simulink model "ctc_sim"  (R2019b)
settings: Solver=VariableStepAuto  StartTime=0.0  StopTime=T  FixedStep=0.001  MaxStep=0.01  RelTol=1e-3
values from neighbouring files (symbols this model uses):
  bsc = 17    [model.mat]    (also in model_data.m)
  d_r = [0.01 0.01 0.01 0.01 0.01 0.01]    [model.mat]    (also in model_data.m = 0.01*ones(6,1))
  Fi_b_z = [0 2.09439510239 4.18879020479 1.0471975512 3.14159265359 5.23598775598]    [model.mat]    (also in model_data.m = [0;2/3;4/3;1/3;3/3;5/3]*pi)
  Kd = 0    [ctc_data.m]
  Ki = 0    [ctc_data.m]
  Kp = 300    [ctc_data.m]
  ksc = 179000    [model.mat]    (also in model_data.m)
  l_r = [0.36 0.36 0.36 0.36 0.36 0.36]    [model.mat]    (also in model_data.m = 0.36*ones(6,1))
  linderiv = 0    [model.mat]    (also in model_data.m)
  O_lb = [0 0 0 0 0 0]    [model.mat]    (also in model_data.m = [0;0;0;0;0;0])
  q_d = out_ik.q'    [ik_run.m]
  qt_d = out_ik.qt'    [ik_run.m]
  qtt_d = out_ik.qtt'    [ik_run.m]
  s = out_ctc.s    [ctc_run.m]
  s_0 = s_d(:,:,1)    [ctc_run.m]    (also in iff_run.m)
  t_d = out_ik.t'    [ik_run.m]
  v_0 = v_d(:,:,1)    [ctc_run.m]    (also in iff_run.m)
  w_lb = 0.195    [model.mat]    (also in model_data.m)
  W_lb = 0.205    [model.mat]    (also in model_data.m)
  w_ub = 0.195    [model.mat]    (also in model_data.m)
  W_ub = 0.205    [model.mat]    (also in model_data.m)
undefined symbols (not defined in the file or in its folder): X, Y, Z
libraries: nesl_utility x280, sm_lib x208, dspindex x30, simulink_extras x18
(part 1 of 13)
settings Model: Creator=Vojta  LastModifiedBy=Tom
settings ExplorerConfigSet: InternalSimMechanicsExplorerSettings="<ExplorerConfiguration><canonicalview>default</canonicalview><AnimationSetting><BasePlaybackSpeed>1.0</BasePlaybackSpeed><PlaybackSpeedFactor>1.0</PlaybackSpeedFactor></AnimationSetting><TilePanel><TileInfo><Tiles Columns=\"1\" Count=\"1\" Rows=\"1\"><Column Weight=\"1\"/><Row Weight=\"1\"/><Tile Height=\"1\" Width=\"1\" X=\"0\" Y=\"0\"/></Tiles></TileInfo><SceneInfo><SceneViewer><BGColor><R>0.800000011920928955</R><G>0.800000011920928955</G><B>0.800000011920928955</B></BGColor><Camera><DoPerspective>off</DoPerspective><Position><X>0.685097738431936554</X><Y>0.708411390405585983</Y><Z>0.419719831436795587</Z></Position><Center><X>-5.89655776053188418e-05</X><Y>-0.000501993352412410943</Y><Z>0.252381535522246514</Z></Center><Up><X>-0.109250379592686409</X><Y>-0.127120209843101351</Y><Z>0.985852325050917688</Z></Up><ViewLimDist>1</ViewLimDist><YLim>0.288930054247379331</YLim><XLim>0.560223444501202317</XLim></Camera></SceneViewer></SceneInfo></TilePanel><MechEditorPanel><Cameras/><GfxPanelCameraMap/><VideoCreator><PlaybackSpeedRatio>1.0</PlaybackSpeedRatio><FrameRate>30</FrameRate><VideoFormat>Motion JPEG AVI</VideoFormat><FrameSize>auto</FrameSize></VideoCreator></MechEditorPanel></ExplorerConfiguration>"

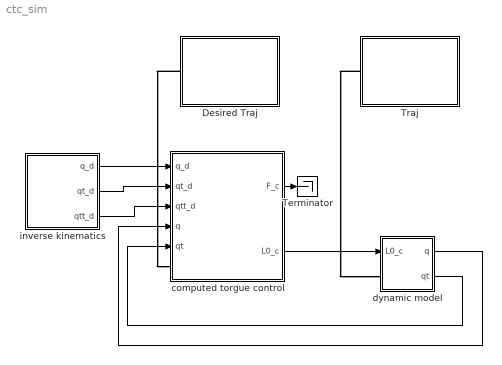
== system ctc_sim ==
  Desired Traj : Subsystem
  Terminator : Terminator
  Traj : Subsystem
  computed torgue control : Subsystem
  dynamic model : Subsystem
  inverse kinematics : Subsystem
  wires:
  inverse kinematics/1(q_d) -> computed torgue control/1(q_d)
  inverse kinematics/2(qt_d) -> computed torgue control/2(qt_d)
  inverse kinematics/3(qtt_d) -> computed torgue control/3(qtt_d)
  dynamic model/2(qt) -> computed torgue control/5(qt)
  dynamic model/1(q) -> computed torgue control/4(q)
  computed torgue control/2(L0_c) -> dynamic model/1(L0_c)
  computed torgue control/1(F_c) -> Terminator/1
  connections:
  Desired Traj/LConn1 -- computed torgue control/LConn1
  Traj/LConn1 -- dynamic model/LConn1

== system ctc_sim/Desired Traj ==
  Angular vels : Scope  NumInputPorts=3
  Mux2 : Mux  Inputs=3
  PS-Simulink Converter{,1..9} (10 alike) : nesl_utility/PS-Simulink Converter  PhysicalDomain=network_engine_domain  SubClassName=ps_output  LeftPortType=input  RightPortType=output  PseudoPeriodic=off  Frequencies=[]  Unit=inherit  AffineConversion=off
  To Workspace2 : ToWorkspace  VariableName=quat_d  SaveFormat=Timeseries  SampleTime=-1
  To Workspace3 : ToWorkspace  VariableName=displacement_d  SaveFormat=Timeseries  SampleTime=-1
  Transform Sensor : sm_lib/Frames and Transforms/Transform Sensor  MeasurementFrame=World  SenseAngle=off  SenseAxis=off  SenseAngle1=off  SenseAngle2=off  SenseAngle3=off  SenseQ=on  SenseR=off  SenseOmegaX=on  SenseOmegaY=on  SenseOmegaZ=on  SenseOmega1=off  SenseOmega2=off  SenseOmega3=off  SenseQDot=off  SenseRDot=off  SenseAlphaX=off  SenseAlphaY=off  SenseAlphaZ=off  SenseAlpha1=off  SenseAlpha2=off  SenseAlpha3=off  SenseQDDot=off  SenseRDDot=off  SenseX=on  SenseY=on  SenseZ=on  SenseRad=off  SenseAzim=off  SenseDist=off  SenseInc=off  SenseXDot=on  SenseYDot=on  SenseZDot=on  SenseRadDot=off  SenseAzimDot=off  SenseDistDot=off  SenseIncDot=off  SenseXDDot=off  SenseYDDot=off  SenseZDDot=off  SenseRadDDot=off  SenseAzimDDot=off  SenseDistDDot=off  SenseIncDDot=off
  Translational vel : Scope  NumInputPorts=3
  Translational disp : Scope  NumInputPorts=3
  World Frame : sm_lib/Frames and Transforms/World Frame
  Top CS : PMIOPort  Side=Left
  wires:
  Mux2/1 -> To Workspace3/1
  PS-Simulink Converter6/1 -> Translational vel/1
  PS-Simulink Converter9/1 -> To Workspace2/1
  PS-Simulink Converter8/1 -> Translational vel/3
  PS-Simulink Converter7/1 -> Translational vel/2
  PS-Simulink Converter5/1 -> Mux2/3, Translational disp/3
  PS-Simulink Converter/1 -> Angular vels/1
  PS-Simulink Converter1/1 -> Angular vels/2
  PS-Simulink Converter3/1 -> Mux2/1, Translational disp/1
  PS-Simulink Converter2/1 -> Angular vels/3
  PS-Simulink Converter4/1 -> Mux2/2, Translational disp/2
  connections:
  Transform Sensor/RConn10 -- PS-Simulink Converter7/LConn1
  World Frame/RConn1 -- Transform Sensor/LConn1
  Transform Sensor/RConn7 -- PS-Simulink Converter4/LConn1
  Transform Sensor/RConn4 -- PS-Simulink Converter1/LConn1
  Transform Sensor/RConn3 -- PS-Simulink Converter/LConn1
  Transform Sensor/RConn6 -- PS-Simulink Converter3/LConn1
  Transform Sensor/RConn9 -- PS-Simulink Converter6/LConn1
  Transform Sensor/RConn5 -- PS-Simulink Converter2/LConn1
  Transform Sensor/RConn11 -- PS-Simulink Converter8/LConn1
  Transform Sensor/RConn8 -- PS-Simulink Converter5/LConn1
  Transform Sensor/RConn2 -- PS-Simulink Converter9/LConn1
  Transform Sensor/RConn1 -- Top CS/RConn1

== system ctc_sim/Traj ==
  Angular vels : Scope  NumInputPorts=3
  Mux2 : Mux  Inputs=3
  PS-Simulink Converter{,1..9} (10 alike) : nesl_utility/PS-Simulink Converter  PhysicalDomain=network_engine_domain  SubClassName=ps_output  LeftPortType=input  RightPortType=output  PseudoPeriodic=off  Frequencies=[]  Unit=inherit  AffineConversion=off
  To Workspace2 : ToWorkspace  VariableName=quat  SaveFormat=Timeseries  SampleTime=-1
  To Workspace3 : ToWorkspace  VariableName=displacement  SaveFormat=Timeseries  SampleTime=-1
  Transform Sensor : sm_lib/Frames and Transforms/Transform Sensor  MeasurementFrame=World  SenseAngle=off  SenseAxis=off  SenseAngle1=off  SenseAngle2=off  SenseAngle3=off  SenseQ=on  SenseR=off  SenseOmegaX=on  SenseOmegaY=on  SenseOmegaZ=on  SenseOmega1=off  SenseOmega2=off  SenseOmega3=off  SenseQDot=off  SenseRDot=off  SenseAlphaX=off  SenseAlphaY=off  SenseAlphaZ=off  SenseAlpha1=off  SenseAlpha2=off  SenseAlpha3=off  SenseQDDot=off  SenseRDDot=off  SenseX=on  SenseY=on  SenseZ=on  SenseRad=off  SenseAzim=off  SenseDist=off  SenseInc=off  SenseXDot=on  SenseYDot=on  SenseZDot=on  SenseRadDot=off  SenseAzimDot=off  SenseDistDot=off  SenseIncDot=off  SenseXDDot=off  SenseYDDot=off  SenseZDDot=off  SenseRadDDot=off  SenseAzimDDot=off  SenseDistDDot=off  SenseIncDDot=off
  Translational vel : Scope  NumInputPorts=3
  Translational disp : Scope  NumInputPorts=3
  World Frame : sm_lib/Frames and Transforms/World Frame
  Top CS : PMIOPort  Side=Left
  wires:
  PS-Simulink Converter4/1 -> Translational disp/2, Mux2/2
  PS-Simulink Converter2/1 -> Angular vels/3
  PS-Simulink Converter3/1 -> Translational disp/1, Mux2/1
  PS-Simulink Converter1/1 -> Angular vels/2
  PS-Simulink Converter/1 -> Angular vels/1
  PS-Simulink Converter5/1 -> Translational disp/3, Mux2/3
  PS-Simulink Converter7/1 -> Translational vel/2
  PS-Simulink Converter8/1 -> Translational vel/3
  PS-Simulink Converter9/1 -> To Workspace2/1
  PS-Simulink Converter6/1 -> Translational vel/1
  Mux2/1 -> To Workspace3/1
  connections:
  Transform Sensor/RConn1 -- Top CS/RConn1
  Transform Sensor/RConn2 -- PS-Simulink Converter9/LConn1
  Transform Sensor/RConn8 -- PS-Simulink Converter5/LConn1
  Transform Sensor/RConn11 -- PS-Simulink Converter8/LConn1
  Transform Sensor/RConn5 -- PS-Simulink Converter2/LConn1
  Transform Sensor/RConn9 -- PS-Simulink Converter6/LConn1
  Transform Sensor/RConn6 -- PS-Simulink Converter3/LConn1
  Transform Sensor/RConn3 -- PS-Simulink Converter/LConn1
  Transform Sensor/RConn4 -- PS-Simulink Converter1/LConn1
  Transform Sensor/RConn7 -- PS-Simulink Converter4/LConn1
  World Frame/RConn1 -- Transform Sensor/LConn1
  Transform Sensor/RConn10 -- PS-Simulink Converter7/LConn1

== system ctc_sim/computed torgue control ==
  q_d : Inport
  qt_d : Inport  Port=2
  qtt_d : Inport  Port=3
  q : Inport  Port=4
  qt : Inport  Port=5
  Constant : Constant  Value=ksc
  Free cable lengths : Subsystem
  To Workspace : ToWorkspace  Commented=on  VariableName=s_ctc  SampleTime=-1
  To Workspace1 : ToWorkspace  Commented=on  VariableName=v_ctc  SampleTime=-1
  To Workspace2 : ToWorkspace  VariableName=F_c  SampleTime=-1
  To Workspace3 : ToWorkspace  VariableName=L0_c  SampleTime=-1
  bases + rods : Subsystem  mask{s_r_0=s_0(:,1:6), v_r_0=v_0(:,1:6), s_ub_0=s_0(:,7), v_ub_0=v_0(:,7)}
  desired cable vectors/ lengths : Subsystem
  "q_d,q -> a_ctc" : Subsystem
  scope F_c : Scope  Commented=on
  scope l_c,d : Scope  Commented=on
  scope q_ctc : Subsystem  Commented=on
  scope qt_ctc : Subsystem  Commented=on
  scope qtt_ctc : Subsystem  Commented=on
  Top CS Desired : PMIOPort  Side=Left
  F_c : Outport
  L0_c : Outport  Port=2
  wires:
  bases + rods/2(v_ctc) -> To Workspace1/1
  q_d/1 -> "q_d,q -> a_ctc"/1(q_d)
  "q_d,q -> a_ctc"/1(q_ctc) -> scope q_ctc/1(in), bases + rods/1(q_ctc)
  "q_d,q -> a_ctc"/3(qtt_ctc) -> scope qtt_ctc/1(in), bases + rods/3(qtt_ctc)
  bases + rods/1(s_ctc) -> To Workspace/1
  "q_d,q -> a_ctc"/2(qt_ctc) -> scope qt_ctc/1(in), bases + rods/2(qt_ctc)
  qt_d/1 -> "q_d,q -> a_ctc"/2(qt_d)
  qtt_d/1 -> "q_d,q -> a_ctc"/3(qtt_d)
  desired cable vectors/ lengths/1(l_c) -> Free cable lengths/1(Desired len), scope l_c,d/1
  q/1 -> "q_d,q -> a_ctc"/4(q)
  qt/1 -> "q_d,q -> a_ctc"/5(qt)
  desired cable vectors/ lengths/2(F_c) -> Free cable lengths/3(Desired F), scope F_c/1, F_c/1, To Workspace2/1
  Constant/1 -> Free cable lengths/2(Specific k)
  Free cable lengths/1(L0(t)) -> To Workspace3/1, L0_c/1
  connections:
  desired cable vectors/ lengths/LConn24 -- desired cable vectors/ lengths/LConn30 -- desired cable vectors/ lengths/LConn14 -- desired cable vectors/ lengths/LConn12 -- bases + rods/RConn11
  bases + rods/RConn3 -- desired cable vectors/ lengths/LConn5 -- desired cable vectors/ lengths/LConn7
  desired cable vectors/ lengths/LConn20 -- desired cable vectors/ lengths/LConn22 -- desired cable vectors/ lengths/LConn26 -- desired cable vectors/ lengths/LConn8 -- bases + rods/RConn9
  bases + rods/RConn5 -- desired cable vectors/ lengths/LConn9 -- desired cable vectors/ lengths/LConn11
  desired cable vectors/ lengths/LConn19 -- desired cable vectors/ lengths/LConn28 -- desired cable vectors/ lengths/LConn17 -- desired cable vectors/ lengths/LConn2 -- bases + rods/RConn4
  desired cable vectors/ lengths/LConn21 -- desired cable vectors/ lengths/LConn23 -- desired cable vectors/ lengths/LConn32 -- desired cable vectors/ lengths/LConn6 -- bases + rods/RConn6
  bases + rods/RConn10 -- desired cable vectors/ lengths/LConn29 -- desired cable vectors/ lengths/LConn31
  desired cable vectors/ lengths/LConn18 -- desired cable vectors/ lengths/LConn34 -- desired cable vectors/ lengths/LConn16 -- desired cable vectors/ lengths/LConn4 -- bases + rods/RConn7
  bases + rods/RConn8 -- desired cable vectors/ lengths/LConn25 -- desired cable vectors/ lengths/LConn27
  desired cable vectors/ lengths/LConn13 -- desired cable vectors/ lengths/LConn36 -- desired cable vectors/ lengths/LConn15 -- desired cable vectors/ lengths/LConn10 -- bases + rods/RConn2
  bases + rods/RConn12 -- desired cable vectors/ lengths/LConn33 -- desired cable vectors/ lengths/LConn35
  bases + rods/RConn1 -- desired cable vectors/ lengths/LConn1 -- desired cable vectors/ lengths/LConn3
  Top CS Desired/RConn1 -- bases + rods/LConn1

== system ctc_sim/dynamic model ==
  L0_c : Inport
  Constant : Constant  Value=ksc
  Real cable forces with spools only : Subsystem
  To Workspace : ToWorkspace  VariableName=l_c  SampleTime=-1
  To Workspace1 : ToWorkspace  VariableName=q  SampleTime=-1
  To Workspace2 : ToWorkspace  VariableName=qt  SampleTime=-1
  cables : Subsystem
  rods + bases : Subsystem  mask{s_r_0=s_0(:,1:6), v_r_0=v_0(:,1:6), s_ub_0=s_0(:,7), v_ub_0=v_0(:,7)}
  "s -> q" : MATLAB Function  TreatAsAtomicUnit=on
  scope l_c : Scope  Commented=on
  "v -> qt" : MATLAB Function  TreatAsAtomicUnit=on
  Top CS : PMIOPort  Side=Left
  q : Outport
  qt : Outport  Port=2
  wires:
  rods + bases/1(s) -> "s -> q"/1(s)
  rods + bases/2(v) -> "v -> qt"/1(v)
  "s -> q"/1(q) -> To Workspace1/1, q/1
  "v -> qt"/1(qt) -> To Workspace2/1, qt/1
  cables/1(l_c) -> Real cable forces with spools only/3(L(t)), To Workspace/1, scope l_c/1
  Real cable forces with spools only/1(Fc(t)) -> cables/1(F_c)
  Constant/1 -> Real cable forces with spools only/2(ksc)
  L0_c/1 -> Real cable forces with spools only/1(L0(t))
  connections:
  rods + bases/RConn1 -- cables/LConn3 -- cables/LConn1
  cables/LConn13 -- cables/LConn15 -- cables/LConn36 -- cables/LConn10 -- rods + bases/RConn2
  rods + bases/RConn3 -- cables/LConn7 -- cables/LConn5
  cables/LConn17 -- cables/LConn19 -- cables/LConn28 -- cables/LConn2 -- rods + bases/RConn4
  rods + bases/RConn5 -- cables/LConn11 -- cables/LConn9
  cables/LConn21 -- cables/LConn23 -- cables/LConn32 -- cables/LConn6 -- rods + bases/RConn6
  cables/LConn16 -- cables/LConn18 -- cables/LConn34 -- cables/LConn4 -- rods + bases/RConn7
  rods + bases/RConn8 -- cables/LConn27 -- cables/LConn25
  cables/LConn20 -- cables/LConn22 -- cables/LConn26 -- cables/LConn8 -- rods + bases/RConn9
  rods + bases/RConn10 -- cables/LConn29 -- cables/LConn31
  cables/LConn14 -- cables/LConn24 -- cables/LConn30 -- cables/LConn12 -- rods + bases/RConn11
  rods + bases/RConn12 -- cables/LConn35 -- cables/LConn33
  Top CS/RConn1 -- rods + bases/LConn1

== system ctc_sim/inverse kinematics ==
  Clock : Clock
  To Workspace : ToWorkspace  VariableName=t  SampleTime=-1
  "t -> q_d" : Subsystem  mask{Q_d=q_d}
  "t -> qt_d" : Subsystem  mask{Q_d=qt_d}
  "t -> qtt_d" : Subsystem  mask{Q_d=qtt_d}
  q_d : Outport
  qt_d : Outport  Port=2
  qtt_d : Outport  Port=3
  wires:
  "t -> q_d"/1(Q_d) -> q_d/1
  Clock/1 -> "t -> qt_d"/1(t), To Workspace/1, "t -> qtt_d"/1(t), "t -> q_d"/1(t)
  "t -> qt_d"/1(Q_d) -> qt_d/1
  "t -> qtt_d"/1(Q_d) -> qtt_d/1

== system ctc_sim/computed torgue control/Free cable lengths ==
  note: 1) actuator length and stiffness neglected
      | 2) damping forces neglected
  Desired len : Inport
  Specific k : Inport  Port=2
  Desired F : Inport  Port=3
  Divide : Product  Inputs=/**
  Sum2 : Sum  Inputs=|++
  L0(t) : Outport
  wires:
  Desired F/1 -> Sum2/1
  Desired len/1 -> Divide/3
  Divide/1 -> L0(t)/1  "L0(t)"
  Sum2/1 -> Divide/1
  Specific k/1 -> Sum2/2, Divide/2

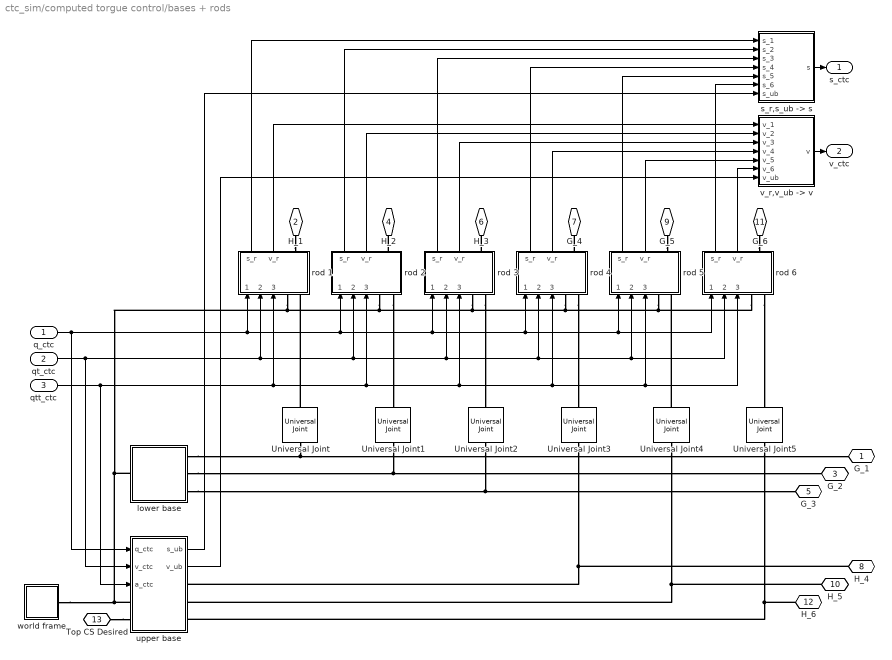
== system ctc_sim/computed torgue control/bases + rods ==
  q_ctc : Inport
  qt_ctc : Inport  Port=2
  qtt_ctc : Inport  Port=3
  Universal Joint{,1..5} (6 alike) : sm_lib/Joints/Universal Joint  JointMode=Normal  SenseConstraintForce=off  SenseConstraintForceX=off  SenseConstraintForceY=off  SenseConstraintForceZ=off  SenseConstraintTorque=off  SenseConstraintTorqueX=off  SenseConstraintTorqueY=off  SenseConstraintTorqueZ=off  SenseTotalForce=off  SenseTotalForceX=off  SenseTotalForceY=off  SenseTotalForceZ=off  SenseTotalTorque=off  SenseTotalTorqueX=off  SenseTotalTorqueY=off  SenseTotalTorqueZ=off  CompositeWrenchDir=FollowerOnBase  CompositeWrenchFrame=BaseFrame  RxEquilibriumPosition=0  RxEquilibriumPositionUnits=deg  RxSpringStiffness=0  RxSpringStiffnessUnits=N*m/deg  RxDampingCoefficient=0  RxDampingCoefficientUnits=N*m/(deg/s)  RxTorqueActuationMode=NoTorque  RxMotionActuationMode=ComputedMotion  RxSensePosition=off  RxSenseVelocity=off  RxSenseAcceleration=off  RxSenseTorqueForce=off  RxSenseLowerLimitTorqueForce=off  RxSenseUpperLimitTorqueForce=off  RxLowerLimitSpecify=off  RxLowerLimitBound=-90  RxLowerLimitBoundUnits=deg  RxLowerLimitStiffness=1e4  RxLowerLimitStiffnessUnits=N*m/deg  RxLowerLimitDamping=10  RxLowerLimitDampingUnits=N*m/(deg/s)  RxLowerLimitTransitionRegionWidth=0.1  RxLowerLimitTransitionRegionWidthUnits=deg  RxUpperLimitSpecify=off  RxUpperLimitBound=90  RxUpperLimitBoundUnits=deg  RxUpperLimitStiffness=1e4  RxUpperLimitStiffnessUnits=N*m/deg  RxUpperLimitDamping=10  RxUpperLimitDampingUnits=N*m/(deg/s)  RxUpperLimitTransitionRegionWidth=0.1  RxUpperLimitTransitionRegionWidthUnits=deg  RxPositionTargetSpecify=off  RxPositionTargetPriority=High  RxPositionTargetValue=0  RxPositionTargetValueUnits=deg  RxVelocityTargetSpecify=off  RxVelocityTargetPriority=High  RxVelocityTargetValue=0  RxVelocityTargetValueUnits=deg/s  RyEquilibriumPosition=0  RyEquilibriumPositionUnits=deg  RySpringStiffness=0  RySpringStiffnessUnits=N*m/deg  RyDampingCoefficient=0  RyDampingCoefficientUnits=N*m/(deg/s)  RyTorqueActuationMode=NoTorque  RyMotionActuationMode=ComputedMotion  RySensePosition=off  RySenseVelocity=off  RySenseAcceleration=off  RySenseTorqueForce=off  RySenseLowerLimitTorqueForce=off  RySenseUpperLimitTorqueForce=off  RyLowerLimitSpecify=off  RyLowerLimitBound=-90  RyLowerLimitBoundUnits=deg  RyLowerLimitStiffness=1e4  RyLowerLimitStiffnessUnits=N*m/deg  RyLowerLimitDamping=10  RyLowerLimitDampingUnits=N*m/(deg/s)  RyLowerLimitTransitionRegionWidth=0.1  RyLowerLimitTransitionRegionWidthUnits=deg  RyUpperLimitSpecify=off  RyUpperLimitBound=90  RyUpperLimitBoundUnits=deg  RyUpperLimitStiffness=1e4  RyUpperLimitStiffnessUnits=N*m/deg  RyUpperLimitDamping=10  RyUpperLimitDampingUnits=N*m/(deg/s)  RyUpperLimitTransitionRegionWidth=0.1  RyUpperLimitTransitionRegionWidthUnits=deg  RyPositionTargetSpecify=off  RyPositionTargetPriority=High  RyPositionTargetValue=0  RyPositionTargetValueUnits=deg  RyVelocityTargetSpecify=off  RyVelocityTargetPriority=High  RyVelocityTargetValue=0  RyVelocityTargetValueUnits=deg/s
      settings: SourceProductName=Simscape Multibody
  lower base : Subsystem
  rod 1 : Subsystem  mask{r=1}
  rod 2 : Subsystem  mask{r=2}
  rod 3 : Subsystem  mask{r=3}
  rod 4 : Subsystem  mask{r=4}
  rod 5 : Subsystem  mask{r=5}
  rod 6 : Subsystem  mask{r=6}
  "s_r,s_ub -> s" : MATLAB Function  TreatAsAtomicUnit=on
  upper base : Subsystem
  "v_r,v_ub -> v" : MATLAB Function  TreatAsAtomicUnit=on
  world frame : Subsystem
  G_1 : PMIOPort  Side=Right
  H_1 : PMIOPort  Port=2  Side=Right
  G_2 : PMIOPort  Port=3  Side=Right
  H_2 : PMIOPort  Port=4  Side=Right
  G_3 : PMIOPort  Port=5  Side=Right
  H_3 : PMIOPort  Port=6  Side=Right
  G_4 : PMIOPort  Port=7  Side=Right
  H_4 : PMIOPort  Port=8  Side=Right
  G_5 : PMIOPort  Port=9  Side=Right
  H_5 : PMIOPort  Port=10  Side=Right
  G_6 : PMIOPort  Port=11  Side=Right
  H_6 : PMIOPort  Port=12  Side=Right
  Top CS Desired : PMIOPort  Port=13  Side=Left
  s_ctc : Outport
  v_ctc : Outport  Port=2
  wires:
  q_ctc/1 -> upper base/1(q_ctc), rod 2/1(q_ctc), rod 3/1(q_ctc), rod 4/1(q_ctc), rod 6/1(q_ctc), rod 5/1(q_ctc), rod 1/1(q_ctc)
  qt_ctc/1 -> upper base/2(v_ctc), rod 2/2(v_ctc), rod 3/2(v_ctc), rod 4/2(v_ctc), rod 6/2(v_ctc), rod 5/2(v_ctc), rod 1/2(v_ctc)
  qtt_ctc/1 -> upper base/3(a_ctc), rod 2/3(a_ctc), rod 3/3(a_ctc), rod 4/3(a_ctc), rod 6/3(a_ctc), rod 5/3(a_ctc), rod 1/3(a_ctc)
  rod 4/1(s_r) -> "s_r,s_ub -> s"/4(s_4)
  rod 3/1(s_r) -> "s_r,s_ub -> s"/3(s_3)
  rod 2/1(s_r) -> "s_r,s_ub -> s"/2(s_2)
  rod 1/1(s_r) -> "s_r,s_ub -> s"/1(s_1)
  "s_r,s_ub -> s"/1(s) -> s_ctc/1
  upper base/1(s_ub) -> "s_r,s_ub -> s"/7(s_ub)
  "v_r,v_ub -> v"/1(v) -> v_ctc/1
  rod 4/2(v_r) -> "v_r,v_ub -> v"/4(v_4)
  rod 3/2(v_r) -> "v_r,v_ub -> v"/3(v_3)
  rod 2/2(v_r) -> "v_r,v_ub -> v"/2(v_2)
  rod 1/2(v_r) -> "v_r,v_ub -> v"/1(v_1)
  upper base/2(v_ub) -> "v_r,v_ub -> v"/7(v_ub)
  rod 5/1(s_r) -> "s_r,s_ub -> s"/5(s_5)
  rod 6/1(s_r) -> "s_r,s_ub -> s"/6(s_6)
  rod 5/2(v_r) -> "v_r,v_ub -> v"/5(v_5)
  rod 6/2(v_r) -> "v_r,v_ub -> v"/6(v_6)
  connections:
  lower base/RConn1 -- Universal Joint/LConn1 -- G_1/RConn1
  lower base/RConn2 -- G_2/RConn1 -- Universal Joint1/LConn1
  lower base/RConn3 -- G_3/RConn1 -- Universal Joint2/LConn1
  Universal Joint3/LConn1 -- H_4/RConn1 -- upper base/RConn1
  Universal Joint4/LConn1 -- H_5/RConn1 -- upper base/RConn2
  H_6/RConn1 -- Universal Joint5/LConn1 -- upper base/RConn3
  H_1/RConn1 -- rod 1/RConn1
  Universal Joint/RConn1 -- rod 1/LConn2
  rod 2/LConn2 -- Universal Joint1/RConn1
  rod 2/RConn1 -- H_2/RConn1
  rod 3/RConn1 -- H_3/RConn1
  world frame/RConn1 -- upper base/LConn1 -- lower base/LConn1 -- rod 1/LConn1 -- rod 2/LConn1 -- rod 3/LConn1 -- rod 4/LConn1 -- rod 6/LConn1 -- rod 5/LConn1
  rod 3/LConn2 -- Universal Joint2/RConn1
  rod 4/LConn2 -- Universal Joint3/RConn1
  rod 4/RConn1 -- G_4/RConn1
  Universal Joint4/RConn1 -- rod 5/LConn2
  G_5/RConn1 -- rod 5/RConn1
  G_6/RConn1 -- rod 6/RConn1
  rod 6/LConn2 -- Universal Joint5/RConn1
  Top CS Desired/RConn1 -- upper base/LConn2

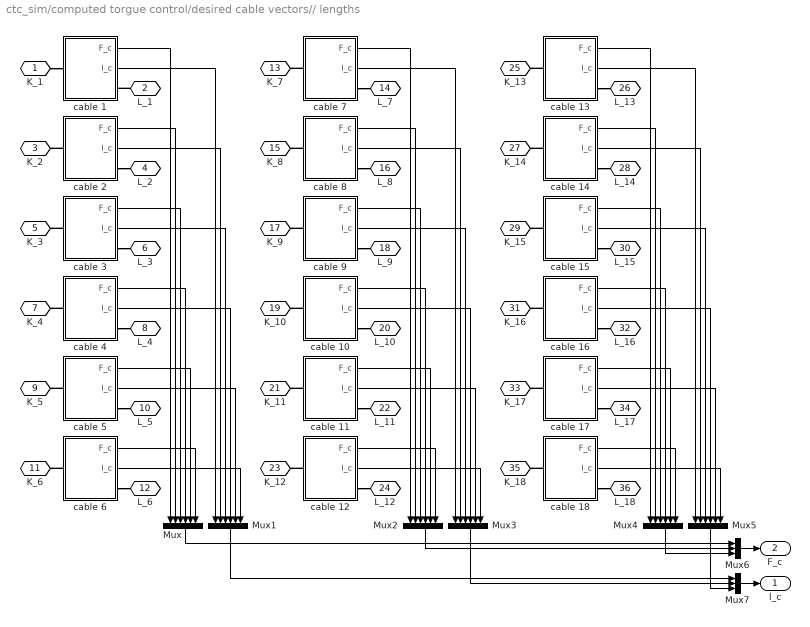
== system ctc_sim/computed torgue control/desired cable vectors// lengths ==
  Mux{,1..5} (6 alike) : Mux  Inputs=6
  Mux6 : Mux  Inputs=3
  Mux7 : Mux  Inputs=3
  cable 1 : Subsystem
  cable 10 : Subsystem
  cable 11 : Subsystem
  cable 12 : Subsystem
  cable 13 : Subsystem
  cable 14 : Subsystem
  cable 15 : Subsystem
  cable 16 : Subsystem
  cable 17 : Subsystem
  cable 18 : Subsystem
  cable 2 : Subsystem
  cable 3 : Subsystem
  cable 4 : Subsystem
  cable 5 : Subsystem
  cable 6 : Subsystem
  cable 7 : Subsystem
  cable 8 : Subsystem
  cable 9 : Subsystem
  K_1 : PMIOPort  Side=Left
  L_1 : PMIOPort  Port=2  Side=Left
  K_2 : PMIOPort  Port=3  Side=Left
  L_2 : PMIOPort  Port=4  Side=Left
  K_3 : PMIOPort  Port=5  Side=Left
  L_3 : PMIOPort  Port=6  Side=Left
  K_4 : PMIOPort  Port=7  Side=Left
  L_4 : PMIOPort  Port=8  Side=Left
  K_5 : PMIOPort  Port=9  Side=Left
  L_5 : PMIOPort  Port=10  Side=Left
  K_6 : PMIOPort  Port=11  Side=Left
  L_6 : PMIOPort  Port=12  Side=Left
  K_7 : PMIOPort  Port=13  Side=Left
  L_7 : PMIOPort  Port=14  Side=Left
  K_8 : PMIOPort  Port=15  Side=Left
  L_8 : PMIOPort  Port=16  Side=Left
  K_9 : PMIOPort  Port=17  Side=Left
  L_9 : PMIOPort  Port=18  Side=Left
  K_10 : PMIOPort  Port=19  Side=Left
  L_10 : PMIOPort  Port=20  Side=Left
  K_11 : PMIOPort  Port=21  Side=Left
  L_11 : PMIOPort  Port=22  Side=Left
  K_12 : PMIOPort  Port=23  Side=Left
  L_12 : PMIOPort  Port=24  Side=Left
  K_13 : PMIOPort  Port=25  Side=Left
  L_13 : PMIOPort  Port=26  Side=Left
  K_14 : PMIOPort  Port=27  Side=Left
  L_14 : PMIOPort  Port=28  Side=Left
  K_15 : PMIOPort  Port=29  Side=Left
  L_15 : PMIOPort  Port=30  Side=Left
  K_16 : PMIOPort  Port=31  Side=Left
  L_16 : PMIOPort  Port=32  Side=Left
  K_17 : PMIOPort  Port=33  Side=Left
  L_17 : PMIOPort  Port=34  Side=Left
  K_18 : PMIOPort  Port=35  Side=Left
  L_18 : PMIOPort  Port=36  Side=Left
  l_c : Outport
  F_c : Outport  Port=2
  wires:
  cable 1/1(F_c) -> Mux/1
  cable 2/1(F_c) -> Mux/2
  cable 3/1(F_c) -> Mux/3
  cable 4/1(F_c) -> Mux/4
  cable 5/1(F_c) -> Mux/5
  cable 6/1(F_c) -> Mux/6
  cable 1/2(l_c) -> Mux1/1
  cable 2/2(l_c) -> Mux1/2
  cable 3/2(l_c) -> Mux1/3
  cable 4/2(l_c) -> Mux1/4
  cable 5/2(l_c) -> Mux1/5
  cable 6/2(l_c) -> Mux1/6
  cable 8/2(l_c) -> Mux3/2
  cable 9/1(F_c) -> Mux2/3
  cable 11/1(F_c) -> Mux2/5
  cable 10/2(l_c) -> Mux3/4
  cable 12/2(l_c) -> Mux3/6
  cable 12/1(F_c) -> Mux2/6
  cable 9/2(l_c) -> Mux3/3
  cable 11/2(l_c) -> Mux3/5
  cable 10/1(F_c) -> Mux2/4
  cable 7/1(F_c) -> Mux2/1
  cable 7/2(l_c) -> Mux3/1
  cable 8/1(F_c) -> Mux2/2
  cable 14/2(l_c) -> Mux5/2
  cable 15/1(F_c) -> Mux4/3
  cable 17/1(F_c) -> Mux4/5
  cable 16/2(l_c) -> Mux5/4
  cable 18/2(l_c) -> Mux5/6
  cable 18/1(F_c) -> Mux4/6
  cable 15/2(l_c) -> Mux5/3
  cable 17/2(l_c) -> Mux5/5
  cable 16/1(F_c) -> Mux4/4
  cable 13/1(F_c) -> Mux4/1
  cable 13/2(l_c) -> Mux5/1
  cable 14/1(F_c) -> Mux4/2
  Mux6/1 -> F_c/1
  Mux/1 -> Mux6/1
  Mux2/1 -> Mux6/2
  Mux4/1 -> Mux6/3
  Mux7/1 -> l_c/1
  Mux1/1 -> Mux7/1
  Mux3/1 -> Mux7/2
  Mux5/1 -> Mux7/3
  connections:
  K_1/RConn1 -- cable 1/LConn1
  L_1/RConn1 -- cable 1/RConn1
  cable 2/RConn1 -- L_2/RConn1
  cable 2/LConn1 -- K_2/RConn1
  cable 3/LConn1 -- K_3/RConn1
  cable 3/RConn1 -- L_3/RConn1
  cable 6/RConn1 -- L_6/RConn1
  cable 4/LConn1 -- K_4/RConn1
  cable 5/RConn1 -- L_5/RConn1
  cable 4/RConn1 -- L_4/RConn1
  cable 6/LConn1 -- K_6/RConn1
  cable 5/LConn1 -- K_5/RConn1
  cable 12/RConn1 -- L_12/RConn1
  cable 11/RConn1 -- L_11/RConn1
  cable 7/LConn1 -- K_7/RConn1
  cable 7/RConn1 -- L_7/RConn1
  cable 12/LConn1 -- K_12/RConn1
  cable 8/LConn1 -- K_8/RConn1
  cable 9/RConn1 -- L_9/RConn1
  cable 10/RConn1 -- L_10/RConn1
  cable 10/LConn1 -- K_10/RConn1
  cable 8/RConn1 -- L_8/RConn1
  cable 9/LConn1 -- K_9/RConn1
  cable 11/LConn1 -- K_11/RConn1
  cable 18/RConn1 -- L_18/RConn1
  cable 17/RConn1 -- L_17/RConn1
  cable 13/LConn1 -- K_13/RConn1
  cable 18/LConn1 -- K_18/RConn1
  cable 13/RConn1 -- L_13/RConn1
  cable 16/RConn1 -- L_16/RConn1
  cable 14/LConn1 -- K_14/RConn1
  cable 14/RConn1 -- L_14/RConn1
  cable 16/LConn1 -- K_16/RConn1
  cable 17/LConn1 -- K_17/RConn1
  cable 15/RConn1 -- L_15/RConn1
  cable 15/LConn1 -- K_15/RConn1

== system ctc_sim/computed torgue control/q_d,q -> a_ctc ==
  q_d : Inport
  qt_d : Inport  Port=2
  qtt_d : Inport  Port=3
  q : Inport  Port=4
  qt : Inport  Port=5
  Gain : Gain  Gain=Kp
  Gain1 : Gain  Gain=Kd
  Gain2 : Gain  Gain=Ki
  Integrator : Integrator
  Sum : Sum  Inputs=+-|
  Sum1 : Sum  Inputs=+-|
  Sum2 : Sum  Inputs=++++
  To Workspace : ToWorkspace  VariableName=e  SampleTime=-1
  q_ctc : Outport
  qt_ctc : Outport  Port=2
  qtt_ctc : Outport  Port=3
  wires:
  q_d/1 -> Sum/1, q_ctc/1
  qt_d/1 -> Sum1/1, qt_ctc/1
  q/1 -> Sum/2
  qt/1 -> Sum1/2
  Sum2/1 -> qtt_ctc/1
  qtt_d/1 -> Sum2/1
  Sum/1 -> Integrator/1, Gain/1, To Workspace/1
  Gain/1 -> Sum2/2
  Sum1/1 -> Gain1/1
  Gain1/1 -> Sum2/3
  Gain2/1 -> Sum2/4
  Integrator/1 -> Gain2/1

== system ctc_sim/computed torgue control/scope q_ctc ==
  in : Inport
  Multiport Selector : dspindex/Multiport Selector  rowsOrCols=Rows  idxCellArray={ 1,2,3,4,5,6}  idxErrMode=Clip Index
  Multiport Selector1 : dspindex/Multiport Selector  rowsOrCols=Rows  idxCellArray={ 7,8,9,10,11,12}  idxErrMode=Clip Index
  Multiport Selector2 : dspindex/Multiport Selector  rowsOrCols=Rows  idxCellArray={ 13,14,15,16,17,18}  idxErrMode=Clip Index
  r = 1-3 : Scope  NumInputPorts=6
  r = 4-6 : Scope  NumInputPorts=6
  ub : Scope  NumInputPorts=6
  wires:
  Multiport Selector/1 -> r = 1-3/1
  Multiport Selector2/2 -> ub/2
  in/1 -> Multiport Selector2/1, Multiport Selector/1, Multiport Selector1/1
  Multiport Selector/2 -> r = 1-3/2
  Multiport Selector1/5 -> r = 4-6/5
  Multiport Selector2/4 -> ub/4
  Multiport Selector/5 -> r = 1-3/5
  Multiport Selector/6 -> r = 1-3/6
  Multiport Selector2/1 -> ub/1
  Multiport Selector/3 -> r = 1-3/3
  Multiport Selector2/5 -> ub/5
  Multiport Selector/4 -> r = 1-3/4
  Multiport Selector1/6 -> r = 4-6/6
  Multiport Selector1/2 -> r = 4-6/2
  Multiport Selector1/4 -> r = 4-6/4
  Multiport Selector1/3 -> r = 4-6/3
  Multiport Selector1/1 -> r = 4-6/1
  Multiport Selector2/3 -> ub/3
  Multiport Selector2/6 -> ub/6

== system ctc_sim/computed torgue control/scope qt_ctc ==
  in : Inport
  Multiport Selector : dspindex/Multiport Selector  rowsOrCols=Rows  idxCellArray={ 1,2,3,4,5,6}  idxErrMode=Clip Index
  Multiport Selector1 : dspindex/Multiport Selector  rowsOrCols=Rows  idxCellArray={ 7,8,9,10,11,12}  idxErrMode=Clip Index
  Multiport Selector2 : dspindex/Multiport Selector  rowsOrCols=Rows  idxCellArray={ 13,14,15,16,17,18}  idxErrMode=Clip Index
  r = 1-3 : Scope  NumInputPorts=6
  r = 4-6 : Scope  NumInputPorts=6
  ub : Scope  NumInputPorts=6
  wires:
  Multiport Selector/1 -> r = 1-3/1
  Multiport Selector2/2 -> ub/2
  in/1 -> Multiport Selector2/1, Multiport Selector/1, Multiport Selector1/1
  Multiport Selector/2 -> r = 1-3/2
  Multiport Selector1/5 -> r = 4-6/5
  Multiport Selector2/4 -> ub/4
  Multiport Selector/5 -> r = 1-3/5
  Multiport Selector/6 -> r = 1-3/6
  Multiport Selector2/1 -> ub/1
  Multiport Selector/3 -> r = 1-3/3
  Multiport Selector2/5 -> ub/5
  Multiport Selector/4 -> r = 1-3/4
  Multiport Selector1/6 -> r = 4-6/6
  Multiport Selector1/2 -> r = 4-6/2
  Multiport Selector1/4 -> r = 4-6/4
  Multiport Selector1/3 -> r = 4-6/3
  Multiport Selector1/1 -> r = 4-6/1
  Multiport Selector2/3 -> ub/3
  Multiport Selector2/6 -> ub/6

== system ctc_sim/computed torgue control/scope qtt_ctc ==
  in : Inport
  Multiport Selector : dspindex/Multiport Selector  rowsOrCols=Rows  idxCellArray={ 1,2,3,4,5,6}  idxErrMode=Clip Index
  Multiport Selector1 : dspindex/Multiport Selector  rowsOrCols=Rows  idxCellArray={ 7,8,9,10,11,12}  idxErrMode=Clip Index
  Multiport Selector2 : dspindex/Multiport Selector  rowsOrCols=Rows  idxCellArray={ 13,14,15,16,17,18}  idxErrMode=Clip Index
  r = 1-3 : Scope  NumInputPorts=6
  r = 4-6 : Scope  NumInputPorts=6
  ub : Scope  NumInputPorts=6
  wires:
  Multiport Selector/1 -> r = 1-3/1
  Multiport Selector2/2 -> ub/2
  in/1 -> Multiport Selector2/1, Multiport Selector/1, Multiport Selector1/1
  Multiport Selector/2 -> r = 1-3/2
  Multiport Selector1/5 -> r = 4-6/5
  Multiport Selector2/4 -> ub/4
  Multiport Selector/5 -> r = 1-3/5
  Multiport Selector/6 -> r = 1-3/6
  Multiport Selector2/1 -> ub/1
  Multiport Selector/3 -> r = 1-3/3
  Multiport Selector2/5 -> ub/5
  Multiport Selector/4 -> r = 1-3/4
  Multiport Selector1/6 -> r = 4-6/6
  Multiport Selector1/2 -> r = 4-6/2
  Multiport Selector1/4 -> r = 4-6/4
  Multiport Selector1/3 -> r = 4-6/3
  Multiport Selector1/1 -> r = 4-6/1
  Multiport Selector2/3 -> ub/3
  Multiport Selector2/6 -> ub/6

== system ctc_sim/dynamic model/Real cable forces with spools only ==
  L0(t) : Inport
  ksc : Inport  Port=2
  L(t) : Inport  Port=3
  Cable specific stiffness : Constant  Value=bsc
  Derivative : Subsystem  mask{LinOn=linderiv, c=1e4}
      mask prompts: LinOn "Switch value (1 for linearization, 0 for simulation):"; c "Derivative constant  Ns/(s+N):"
  Divide : Product  Inputs=*/*
  Divide1 : Product  Inputs=/**
  Scope : Scope
  Scope1 : Scope
  Sum1 : Sum  Inputs=+|+
  Sum3 : Sum  Inputs=|-+
  Fc(t) : Outport
  wires:
  ksc/1 -> Divide1/3
  Sum3/1 -> Divide1/2
  L0(t)/1 -> Sum3/1, Divide/2, Divide1/1
  Derivative/1(Out1) -> Divide/3
  L(t)/1 -> Derivative/1(In1), Sum3/2
  Cable specific stiffness/1 -> Divide/1
  Divide/1 -> Sum1/1, Scope/1  "Damping force"
  Divide1/1 -> Scope1/1, Sum1/2  "Stiffness force"
  Sum1/1 -> Fc(t)/1

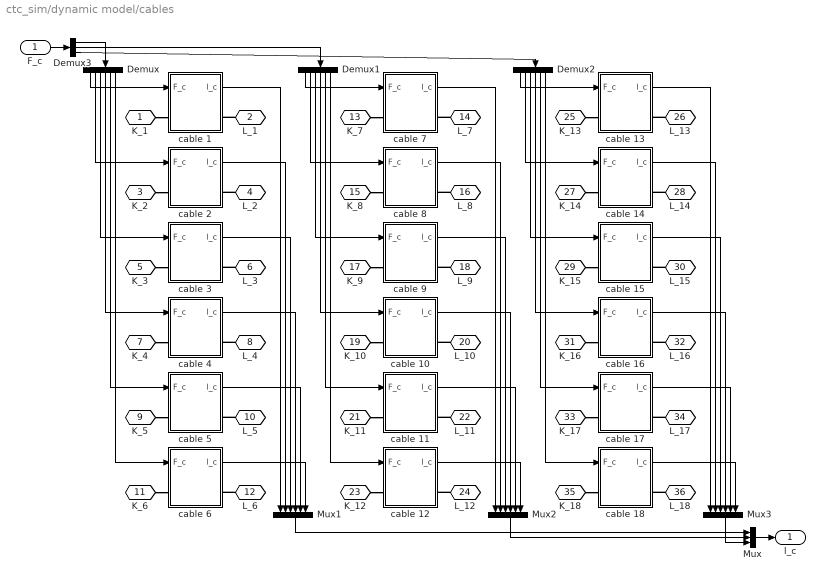
== system ctc_sim/dynamic model/cables ==
  F_c : Inport
  Demux : Demux  Outputs=6
  Demux1 : Demux  Outputs=6
  Demux2 : Demux  Outputs=6
  Demux3 : Demux  Outputs=3
  Mux : Mux  Inputs=3
  Mux1 : Mux  Inputs=6
  Mux2 : Mux  Inputs=6
  Mux3 : Mux  Inputs=6
  cable 1 : Subsystem
  cable 10 : Subsystem
  cable 11 : Subsystem
  cable 12 : Subsystem
  cable 13 : Subsystem
  cable 14 : Subsystem
  cable 15 : Subsystem
  cable 16 : Subsystem
  cable 17 : Subsystem
  cable 18 : Subsystem
  cable 2 : Subsystem
  cable 3 : Subsystem
  cable 4 : Subsystem
  cable 5 : Subsystem
  cable 6 : Subsystem
  cable 7 : Subsystem
  cable 8 : Subsystem
  cable 9 : Subsystem
  K_1 : PMIOPort  Side=Left
  L_1 : PMIOPort  Port=2  Side=Left
  K_2 : PMIOPort  Port=3  Side=Left
  L_2 : PMIOPort  Port=4  Side=Left
  K_3 : PMIOPort  Port=5  Side=Left
  L_3 : PMIOPort  Port=6  Side=Left
  K_4 : PMIOPort  Port=7  Side=Left
  L_4 : PMIOPort  Port=8  Side=Left
  K_5 : PMIOPort  Port=9  Side=Left
  L_5 : PMIOPort  Port=10  Side=Left
  K_6 : PMIOPort  Port=11  Side=Left
  L_6 : PMIOPort  Port=12  Side=Left
  K_7 : PMIOPort  Port=13  Side=Left
  L_7 : PMIOPort  Port=14  Side=Left
  K_8 : PMIOPort  Port=15  Side=Left
  L_8 : PMIOPort  Port=16  Side=Left
  K_9 : PMIOPort  Port=17  Side=Left
  L_9 : PMIOPort  Port=18  Side=Left
  K_10 : PMIOPort  Port=19  Side=Left
  L_10 : PMIOPort  Port=20  Side=Left
  K_11 : PMIOPort  Port=21  Side=Left
  L_11 : PMIOPort  Port=22  Side=Left
  K_12 : PMIOPort  Port=23  Side=Left
  L_12 : PMIOPort  Port=24  Side=Left
  K_13 : PMIOPort  Port=25  Side=Left
  L_13 : PMIOPort  Port=26  Side=Left
  K_14 : PMIOPort  Port=27  Side=Left
  L_14 : PMIOPort  Port=28  Side=Left
  K_15 : PMIOPort  Port=29  Side=Left
  L_15 : PMIOPort  Port=30  Side=Left
  K_16 : PMIOPort  Port=31  Side=Left
  L_16 : PMIOPort  Port=32  Side=Left
  K_17 : PMIOPort  Port=33  Side=Left
  L_17 : PMIOPort  Port=34  Side=Left
  K_18 : PMIOPort  Port=35  Side=Left
  L_18 : PMIOPort  Port=36  Side=Left
  l_c : Outport
  wires:
  F_c/1 -> Demux3/1
  Mux/1 -> l_c/1
  Demux/1 -> cable 1/1(F_c)
  Demux/2 -> cable 2/1(F_c)
  Demux/3 -> cable 3/1(F_c)
  Demux/4 -> cable 4/1(F_c)
  Demux/5 -> cable 5/1(F_c)
  Demux/6 -> cable 6/1(F_c)
  cable 1/1(l_c) -> Mux1/1
  cable 2/1(l_c) -> Mux1/2
  cable 3/1(l_c) -> Mux1/3
  cable 4/1(l_c) -> Mux1/4
  cable 5/1(l_c) -> Mux1/5
  cable 6/1(l_c) -> Mux1/6
  cable 11/1(l_c) -> Mux2/5
  cable 8/1(l_c) -> Mux2/2
  Demux1/5 -> cable 11/1(F_c)
  Demux1/3 -> cable 9/1(F_c)
  Demux1/1 -> cable 7/1(F_c)
  Demux1/4 -> cable 10/1(F_c)
  cable 9/1(l_c) -> Mux2/3
  Demux1/2 -> cable 8/1(F_c)
  Demux1/6 -> cable 12/1(F_c)
  cable 7/1(l_c) -> Mux2/1
  cable 10/1(l_c) -> Mux2/4
  cable 12/1(l_c) -> Mux2/6
  cable 17/1(l_c) -> Mux3/5
  cable 14/1(l_c) -> Mux3/2
  Demux2/5 -> cable 17/1(F_c)
  Demux2/3 -> cable 15/1(F_c)
  Demux2/1 -> cable 13/1(F_c)
  Demux2/4 -> cable 16/1(F_c)
  cable 15/1(l_c) -> Mux3/3
  Demux2/2 -> cable 14/1(F_c)
  Demux2/6 -> cable 18/1(F_c)
  cable 13/1(l_c) -> Mux3/1
  cable 16/1(l_c) -> Mux3/4
  cable 18/1(l_c) -> Mux3/6
  Demux3/1 -> Demux/1
  Demux3/2 -> Demux1/1
  Demux3/3 -> Demux2/1
  Mux1/1 -> Mux/1
  Mux2/1 -> Mux/2
  Mux3/1 -> Mux/3
  connections:
  K_2/RConn1 -- cable 2/LConn1
  L_2/RConn1 -- cable 2/RConn1
  K_3/RConn1 -- cable 3/LConn1
  L_3/RConn1 -- cable 3/RConn1
  K_1/RConn1 -- cable 1/LConn1
  L_1/RConn1 -- cable 1/RConn1
  K_5/RConn1 -- cable 5/LConn1
  L_4/RConn1 -- cable 4/RConn1
  L_5/RConn1 -- cable 5/RConn1
  K_6/RConn1 -- cable 6/LConn1
  L_6/RConn1 -- cable 6/RConn1
  K_4/RConn1 -- cable 4/LConn1
  L_12/RConn1 -- cable 12/RConn1
  L_7/RConn1 -- cable 7/RConn1
  L_9/RConn1 -- cable 9/RConn1
  K_9/RConn1 -- cable 9/LConn1
  K_10/RConn1 -- cable 10/LConn1
  L_11/RConn1 -- cable 11/RConn1
  K_11/RConn1 -- cable 11/LConn1
  K_8/RConn1 -- cable 8/LConn1
  K_7/RConn1 -- cable 7/LConn1
  L_8/RConn1 -- cable 8/RConn1
  K_12/RConn1 -- cable 12/LConn1
  L_10/RConn1 -- cable 10/RConn1
  L_15/RConn1 -- cable 15/RConn1
  L_13/RConn1 -- cable 13/RConn1
  K_16/RConn1 -- cable 16/LConn1
  K_13/RConn1 -- cable 13/LConn1
  L_17/RConn1 -- cable 17/RConn1
  K_14/RConn1 -- cable 14/LConn1
  L_16/RConn1 -- cable 16/RConn1
  K_15/RConn1 -- cable 15/LConn1
  L_18/RConn1 -- cable 18/RConn1
  L_14/RConn1 -- cable 14/RConn1
  K_18/RConn1 -- cable 18/LConn1
  K_17/RConn1 -- cable 17/LConn1

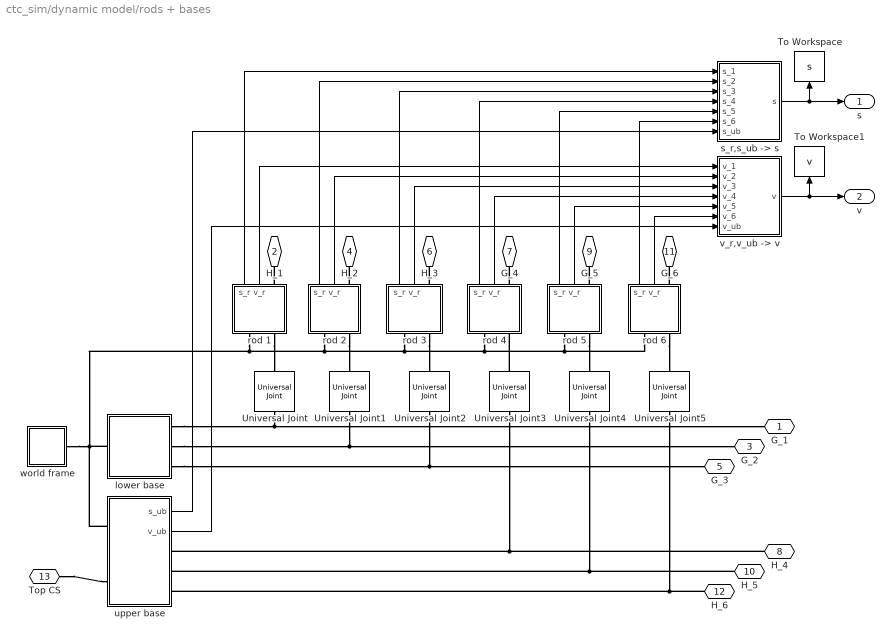
== system ctc_sim/dynamic model/rods + bases ==
  To Workspace : ToWorkspace  VariableName=s  SampleTime=-1
  To Workspace1 : ToWorkspace  VariableName=v  SampleTime=-1
  Universal Joint{,1..5} (6 alike) : sm_lib/Joints/Universal Joint  JointMode=Normal  SenseConstraintForce=off  SenseConstraintForceX=off  SenseConstraintForceY=off  SenseConstraintForceZ=off  SenseConstraintTorque=off  SenseConstraintTorqueX=off  SenseConstraintTorqueY=off  SenseConstraintTorqueZ=off  SenseTotalForce=off  SenseTotalForceX=off  SenseTotalForceY=off  SenseTotalForceZ=off  SenseTotalTorque=off  SenseTotalTorqueX=off  SenseTotalTorqueY=off  SenseTotalTorqueZ=off  CompositeWrenchDir=FollowerOnBase  CompositeWrenchFrame=BaseFrame  RxEquilibriumPosition=0  RxEquilibriumPositionUnits=deg  RxSpringStiffness=0  RxSpringStiffnessUnits=N*m/deg  RxDampingCoefficient=0  RxDampingCoefficientUnits=N*m/(deg/s)  RxTorqueActuationMode=NoTorque  RxMotionActuationMode=ComputedMotion  RxSensePosition=off  RxSenseVelocity=off  RxSenseAcceleration=off  RxSenseTorqueForce=off  RxSenseLowerLimitTorqueForce=off  RxSenseUpperLimitTorqueForce=off  RxLowerLimitSpecify=off  RxLowerLimitBound=-90  RxLowerLimitBoundUnits=deg  RxLowerLimitStiffness=1e4  RxLowerLimitStiffnessUnits=N*m/deg  RxLowerLimitDamping=10  RxLowerLimitDampingUnits=N*m/(deg/s)  RxLowerLimitTransitionRegionWidth=0.1  RxLowerLimitTransitionRegionWidthUnits=deg  RxUpperLimitSpecify=off  RxUpperLimitBound=90  RxUpperLimitBoundUnits=deg  RxUpperLimitStiffness=1e4  RxUpperLimitStiffnessUnits=N*m/deg  RxUpperLimitDamping=10  RxUpperLimitDampingUnits=N*m/(deg/s)  RxUpperLimitTransitionRegionWidth=0.1  RxUpperLimitTransitionRegionWidthUnits=deg  RxPositionTargetSpecify=off  RxPositionTargetPriority=High  RxPositionTargetValue=0  RxPositionTargetValueUnits=deg  RxVelocityTargetSpecify=off  RxVelocityTargetPriority=High  RxVelocityTargetValue=0  RxVelocityTargetValueUnits=deg/s  RyEquilibriumPosition=0  RyEquilibriumPositionUnits=deg  RySpringStiffness=0  RySpringStiffnessUnits=N*m/deg  RyDampingCoefficient=0  RyDampingCoefficientUnits=N*m/(deg/s)  RyTorqueActuationMode=NoTorque  RyMotionActuationMode=ComputedMotion  RySensePosition=off  RySenseVelocity=off  RySenseAcceleration=off  RySenseTorqueForce=off  RySenseLowerLimitTorqueForce=off  RySenseUpperLimitTorqueForce=off  RyLowerLimitSpecify=off  RyLowerLimitBound=-90  RyLowerLimitBoundUnits=deg  RyLowerLimitStiffness=1e4  RyLowerLimitStiffnessUnits=N*m/deg  RyLowerLimitDamping=10  RyLowerLimitDampingUnits=N*m/(deg/s)  RyLowerLimitTransitionRegionWidth=0.1  RyLowerLimitTransitionRegionWidthUnits=deg  RyUpperLimitSpecify=off  RyUpperLimitBound=90  RyUpperLimitBoundUnits=deg  RyUpperLimitStiffness=1e4  RyUpperLimitStiffnessUnits=N*m/deg  RyUpperLimitDamping=10  RyUpperLimitDampingUnits=N*m/(deg/s)  RyUpperLimitTransitionRegionWidth=0.1  RyUpperLimitTransitionRegionWidthUnits=deg  RyPositionTargetSpecify=off  RyPositionTargetPriority=High  RyPositionTargetValue=0  RyPositionTargetValueUnits=deg  RyVelocityTargetSpecify=off  RyVelocityTargetPriority=High  RyVelocityTargetValue=0  RyVelocityTargetValueUnits=deg/s
      settings: SourceProductName=Simscape Multibody
  lower base : Subsystem
  rod 1 : Subsystem  mask{r=1}
  rod 2 : Subsystem  mask{r=2}
  rod 3 : Subsystem  mask{r=3}
  rod 4 : Subsystem  mask{r=4}
  rod 5 : Subsystem  mask{r=5}
  rod 6 : Subsystem  mask{r=6}
  "s_r,s_ub -> s" : MATLAB Function  TreatAsAtomicUnit=on
  upper base : Subsystem
  "v_r,v_ub -> v" : MATLAB Function  TreatAsAtomicUnit=on
  world frame : Subsystem
  G_1 : PMIOPort  Side=Right
  H_1 : PMIOPort  Port=2  Side=Right
  G_2 : PMIOPort  Port=3  Side=Right
  H_2 : PMIOPort  Port=4  Side=Right
  G_3 : PMIOPort  Port=5  Side=Right
  H_3 : PMIOPort  Port=6  Side=Right
  G_4 : PMIOPort  Port=7  Side=Right
  H_4 : PMIOPort  Port=8  Side=Right
  G_5 : PMIOPort  Port=9  Side=Right
  H_5 : PMIOPort  Port=10  Side=Right
  G_6 : PMIOPort  Port=11  Side=Right
  H_6 : PMIOPort  Port=12  Side=Right
  Top CS : PMIOPort  Port=13  Side=Left
  s : Outport
  v : Outport  Port=2
  wires:
  rod 1/1(s_r) -> "s_r,s_ub -> s"/1(s_1)
  upper base/1(s_ub) -> "s_r,s_ub -> s"/7(s_ub)
  "v_r,v_ub -> v"/1(v) -> To Workspace1/1, v/1
  rod 1/2(v_r) -> "v_r,v_ub -> v"/1(v_1)
  upper base/2(v_ub) -> "v_r,v_ub -> v"/7(v_ub)
  rod 2/2(v_r) -> "v_r,v_ub -> v"/2(v_2)
  rod 2/1(s_r) -> "s_r,s_ub -> s"/2(s_2)
  rod 3/2(v_r) -> "v_r,v_ub -> v"/3(v_3)
  rod 3/1(s_r) -> "s_r,s_ub -> s"/3(s_3)
  rod 4/2(v_r) -> "v_r,v_ub -> v"/4(v_4)
  rod 4/1(s_r) -> "s_r,s_ub -> s"/4(s_4)
  rod 5/1(s_r) -> "s_r,s_ub -> s"/5(s_5)
  rod 5/2(v_r) -> "v_r,v_ub -> v"/5(v_5)
  rod 6/2(v_r) -> "v_r,v_ub -> v"/6(v_6)
  rod 6/1(s_r) -> "s_r,s_ub -> s"/6(s_6)
  "s_r,s_ub -> s"/1(s) -> To Workspace/1, s/1
  connections:
  lower base/RConn1 -- Universal Joint/LConn1 -- G_1/RConn1
  lower base/RConn2 -- G_2/RConn1 -- Universal Joint1/LConn1
  lower base/RConn3 -- G_3/RConn1 -- Universal Joint2/LConn1
  Universal Joint3/LConn1 -- H_4/RConn1 -- upper base/RConn1
  Universal Joint4/LConn1 -- H_5/RConn1 -- upper base/RConn2
  H_6/RConn1 -- Universal Joint5/LConn1 -- upper base/RConn3
  rod 1/RConn1 -- H_1/RConn1
  rod 1/LConn2 -- Universal Joint/RConn1
  world frame/RConn1 -- rod 3/LConn1 -- rod 6/LConn1 -- rod 5/LConn1 -- rod 4/LConn1 -- rod 2/LConn1 -- rod 1/LConn1 -- upper base/LConn1 -- lower base/LConn1
  rod 2/RConn1 -- H_2/RConn1
  rod 2/LConn2 -- Universal Joint1/RConn1
  rod 3/LConn2 -- Universal Joint2/RConn1
  rod 3/RConn1 -- H_3/RConn1
  rod 4/RConn1 -- G_4/RConn1
  Universal Joint3/RConn1 -- rod 4/LConn2
  rod 5/RConn1 -- G_5/RConn1
  rod 5/LConn2 -- Universal Joint4/RConn1
  rod 6/RConn1 -- G_6/RConn1
  rod 6/LConn2 -- Universal Joint5/RConn1
  Top CS/RConn1 -- upper base/LConn2

== system ctc_sim/inverse kinematics/t -> q_d ==
  t : Inport
  Mux : Mux  Inputs=7
  rod 1 : Subsystem  mask{r=1}
  rod 2 : Subsystem  mask{r=2}
  rod 3 : Subsystem  mask{r=3}
  rod 4 : Subsystem  mask{r=4}
  rod 5 : Subsystem  mask{r=5}
  rod 6 : Subsystem  mask{r=6}
  upper base : Subsystem
  Q_d : Outport
  wires:
  t/1 -> rod 4/1(t), rod 3/1(t), rod 2/1(t), rod 1/1(t), rod 5/1(t), rod 6/1(t), upper base/1(t)
  rod 2/1(Q_r,d) -> Mux/2
  Mux/1 -> Q_d/1
  rod 4/1(Q_r,d) -> Mux/4
  rod 5/1(Q_r,d) -> Mux/5
  rod 3/1(Q_r,d) -> Mux/3
  rod 1/1(Q_r,d) -> Mux/1
  upper base/1(Q_ub,d) -> Mux/7
  rod 6/1(Q_r,d) -> Mux/6

== system ctc_sim/inverse kinematics/t -> qt_d ==
  t : Inport
  Mux : Mux  Inputs=7
  rod 1 : Subsystem  mask{r=1}
  rod 2 : Subsystem  mask{r=2}
  rod 3 : Subsystem  mask{r=3}
  rod 4 : Subsystem  mask{r=4}
  rod 5 : Subsystem  mask{r=5}
  rod 6 : Subsystem  mask{r=6}
  upper base : Subsystem
  Q_d : Outport
  wires:
  t/1 -> rod 4/1(t), rod 3/1(t), rod 2/1(t), rod 1/1(t), rod 5/1(t), rod 6/1(t), upper base/1(t)
  rod 2/1(Q_r,d) -> Mux/2
  Mux/1 -> Q_d/1
  rod 4/1(Q_r,d) -> Mux/4
  rod 5/1(Q_r,d) -> Mux/5
  rod 3/1(Q_r,d) -> Mux/3
  rod 1/1(Q_r,d) -> Mux/1
  upper base/1(Q_ub,d) -> Mux/7
  rod 6/1(Q_r,d) -> Mux/6

== system ctc_sim/inverse kinematics/t -> qtt_d ==
  t : Inport
  Mux : Mux  Inputs=7
  rod 1 : Subsystem  mask{r=1}
  rod 2 : Subsystem  mask{r=2}
  rod 3 : Subsystem  mask{r=3}
  rod 4 : Subsystem  mask{r=4}
  rod 5 : Subsystem  mask{r=5}
  rod 6 : Subsystem  mask{r=6}
  upper base : Subsystem
  Q_d : Outport
  wires:
  t/1 -> rod 4/1(t), rod 3/1(t), rod 2/1(t), rod 1/1(t), rod 5/1(t), rod 6/1(t), upper base/1(t)
  rod 2/1(Q_r,d) -> Mux/2
  Mux/1 -> Q_d/1
  rod 4/1(Q_r,d) -> Mux/4
  rod 5/1(Q_r,d) -> Mux/5
  rod 3/1(Q_r,d) -> Mux/3
  rod 1/1(Q_r,d) -> Mux/1
  upper base/1(Q_ub,d) -> Mux/7
  rod 6/1(Q_r,d) -> Mux/6

== system ctc_sim/computed torgue control/bases + rods/lower base ==
  "O_lb -> G_1" : Subsystem
  "O_lb -> G_2" : Subsystem
  "O_lb -> G_3" : Subsystem
  body_lb : sm_lib/Body Elements/Extruded Solid  GraphicAmbientColor=[0.15 0.15 0.15 1.0]  BasedOnType=Density  CenterOfMass=[0 0 0]  CenterOfMassUnits=m  GraphicDiffuseColor=ctc_color  ExtrusionCrossSection=[1 1; -1 1; -1 -1; 1 -1]  ExtrusionCrossSectionUnits=m  Density=Ro_lb  DensityUnits=kg/m^3  DoExposeReferenceFrame=on  GraphicEmissiveColor=[0.0 0.0 0.0 1.0]  ExportEntireGeometry=off  ExtrusionLength=t_lb  ExtrusionLengthUnits=m  ExtrusionType=Regular  SerializedFrames=<Frames/>  MarkerShape=Sphere  MarkerSize=10  GraphicType=FromGeometry  InertiaType=CalculateFromGeometry  Mass=1  MassUnits=kg  MomentsOfInertia=[1 1 1]  MomentsOfInertiaUnits=kg*m^2  PolygonNumSides=6  GraphicOpacity=ctc_opacity  PolygonOuterRadius=(W_lb/2)/cosd(30)  PolygonOuterRadiusUnits=m  ProductsOfInertia=[0 0 0]  ProductsOfInertiaUnits=kg*m^2  GraphicShininess=75  GraphicSpecularColor=[0.5 0.5 0.5 1.0]  GraphicVisPropType=SimpleVisualProperties
      settings: SourceProductName=Simscape Multibody
  "wf -> O_lb" : Subsystem
  G_1 : PMIOPort  Side=Right
  G_2 : PMIOPort  Port=2  Side=Right
  G_3 : PMIOPort  Port=3  Side=Right
  wf : PMIOPort  Port=4  Side=Left
  connections:
  wf/RConn1 -- "wf -> O_lb"/LConn1
  "wf -> O_lb"/RConn1 -- "O_lb -> G_3"/LConn1 -- "O_lb -> G_2"/LConn1 -- body_lb/RConn1 -- "O_lb -> G_1"/LConn1
  G_1/RConn1 -- "O_lb -> G_1"/RConn1
  G_2/RConn1 -- "O_lb -> G_2"/RConn1
  "O_lb -> G_3"/RConn1 -- G_3/RConn1
